simulink model "analise_pi_d"  (R2025a)
settings: Solver=VariableStepAuto  StartTime=0.0  StopTime=150  RelTol=1e-3
values from neighbouring files (symbols this model uses):
  alpha = 0.1    [simulink_constants.m]
  Delay = 0.1    [simulink_constants.m]
  kp = 10    [simulink_constants.m]
  Nm = 10^(-5)    (= 1e-05)    [simulink_constants.m]
  Np = 10^(-9)    (= 1e-09)    [simulink_constants.m]
  td = 0.05    [simulink_constants.m]
  ti = 0.17    [simulink_constants.m]
  Ts = 0.5    [filtro.m]    (also in simulink_constants.m = 0.02; teste2.m)
  Ubar = 5    [simulink_constants.m]
  Ybar = 3.47    [simulink_constants.m]
libraries: simulink x2, cstblocks x1
settings Model: Creator=joaof  LastModifiedBy=joaof

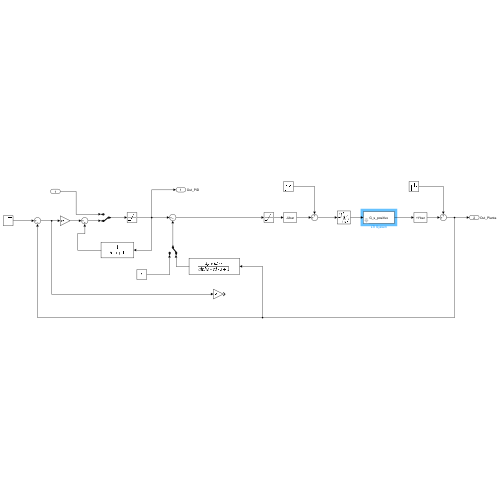
[thumbnail: Simulink's stored preview of the top-level diagram]
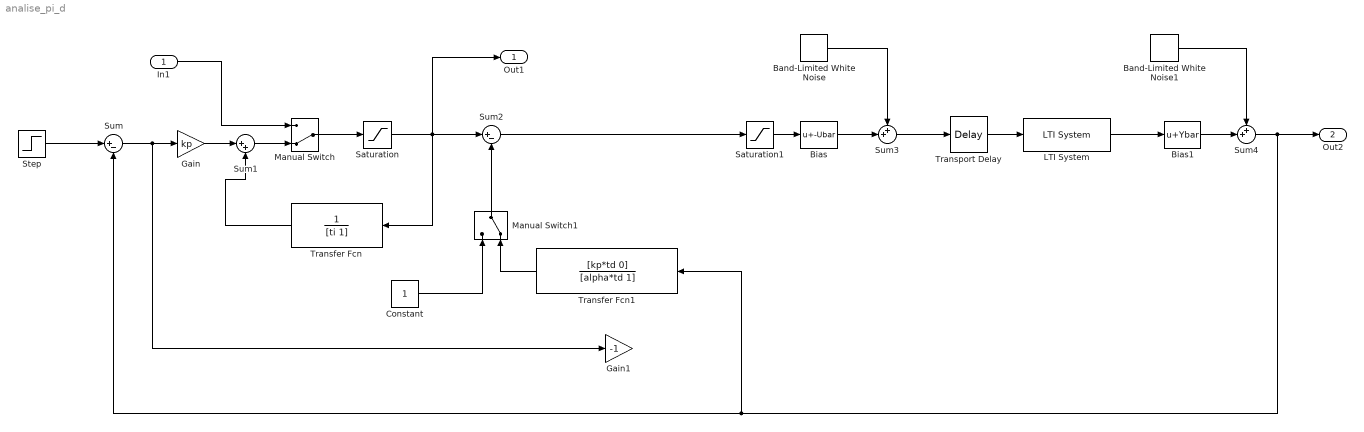
== system analise_pi_d ==
  In1 : Inport
  Band-Limited White Noise : simulink/Sources/Band-Limited White Noise  Cov=[Np]  Ts=Ts  seed=[23341]
  Band-Limited White Noise1 : simulink/Sources/Band-Limited White Noise  Cov=[Nm]  Ts=Ts  seed=[23341]
  Bias : Bias  Bias=-Ubar  SaturateOnIntegerOverflow=off
  Bias1 : Bias  Bias=Ybar  SaturateOnIntegerOverflow=off
  Constant : Constant
  Gain : Gain  Gain=kp
  Gain1 : Gain  Gain=-1
  LTI System : cstblocks/LTI System  sys=G_s_positivo  IC=[]  PadeOrder=0
  Manual Switch : ManualSwitch  CurrentSetting=0
  Manual Switch1 : ManualSwitch  CurrentSetting=0
  Saturation : Saturate  UpperLimit=5  LowerLimit=-5
  Saturation1 : Saturate  UpperLimit=5  LowerLimit=-5
  Step : Step  Before=0.1  After=2.5  SampleTime=0
  Sum : Sum  Inputs=|+-
  Sum1 : Sum  Inputs=|++
  Sum2 : Sum  Inputs=|+-
  Sum3 : Sum  Inputs=++|
  Sum4 : Sum  Inputs=++|
  Transfer Fcn : TransferFcn  Denominator=[ti 1]
  Transfer Fcn1 : TransferFcn  Numerator=[kp*td 0]  Denominator=[alpha*td 1]
  Transport Delay : TransportDelay  DelayTime=Delay
  Out1 : Outport  SignalName=Out_PID
  Out2 : Outport  Port=2  SignalName=Out_Planta
  wires:
  Step/1 -> Sum/1
  Sum/1 -> Gain1/1, Gain/1
  Gain/1 -> Sum1/1
  In1/1 -> Manual Switch/1
  Sum1/1 -> Manual Switch/2
  Transfer Fcn/1 -> Sum1/2
  Manual Switch/1 -> Saturation/1
  Saturation/1 -> Out1/1, Transfer Fcn/1, Sum2/1
  Constant/1 -> Manual Switch1/1
  Transfer Fcn1/1 -> Manual Switch1/2
  Manual Switch1/1 -> Sum2/2
  Saturation1/1 -> Bias/1
  Bias/1 -> Sum3/2
  Band-Limited White Noise/1 -> Sum3/1
  Sum3/1 -> Transport Delay/1
  Transport Delay/1 -> LTI System/1
  LTI System/1 -> Bias1/1
  Bias1/1 -> Sum4/2
  Band-Limited White Noise1/1 -> Sum4/1
  Sum4/1 -> Transfer Fcn1/1, Sum/2, Out2/1
  Sum2/1 -> Saturation1/1
